simulink model "F16ASYM_ControlledFAST"  (R2012b)
settings: Solver=ode4  SolverMode=SingleTasking  StartTime=0.0  StopTime=inf  FixedStep=T_sim  RelTol=1e-3
InitFcn:
  | mex nlplantASYM.c
values from neighbouring files (symbols this model uses):
  T_sim = 0.02    [RUN_ME.m]
undefined symbols (not defined in the file or in its folder): B, dLEF, Earth, fi_flag_Simulink, k_B, latitude, longitude, m, m_B, Model_used_flag, rad, s, sigbuilder_block, trim_control, trim_state, trim_throttle, WGS84
libraries: F16_Actuator_Library x14, simulink_extras x9, aerolibatmos2 x3, aerolibtransform2 x3, aerolibfltsims x3, aerolibconvert2 x2, dspmtrx3 x1, qcatlib x1, aerolibasang x1, aerolibanimutils x1, aerolibconvert x1, aerolibobsolete x1
(part 1 of 2)
settings Model: SimulationMode=accelerator  Creator=David  LastModifiedBy=David
settings DataIOCC: SaveOutput=off  SignalLogging=off  DSMLogging=off  SaveTime=off

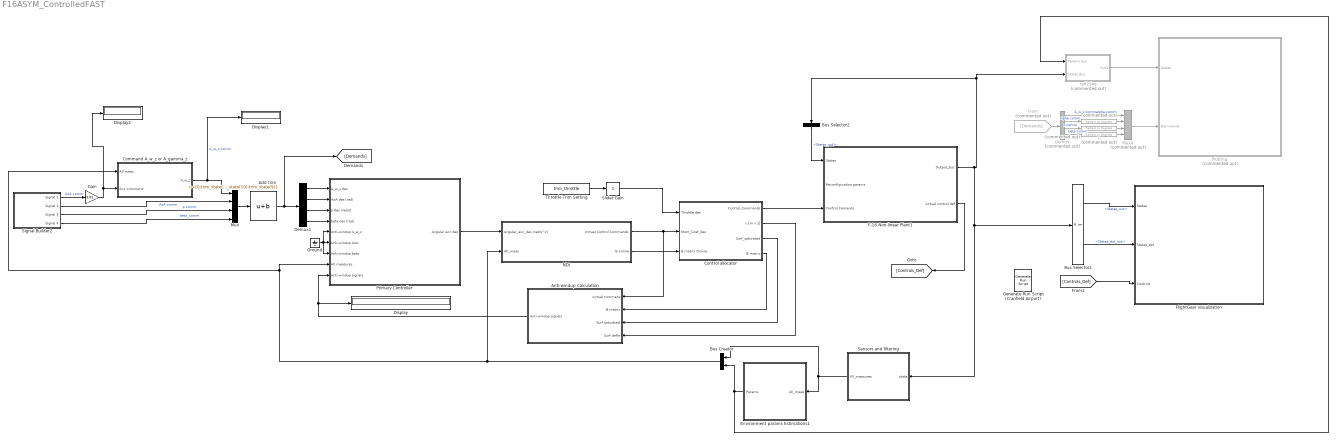
== system F16ASYM_ControlledFAST ==
  "  " : simulink_extras/Transformations/Radians to Degrees  Commented=on
  "  1" : simulink_extras/Transformations/Radians to Degrees  Commented=on
  "  2" : simulink_extras/Transformations/Radians to Degrees  Commented=on
  Add trim : Bias  Bias=[0;trim_state(8);trim_state(10);trim_state(9)]
  Anti-windup Calculation : Subsystem
  Bus Creator : BusCreator  Inputs=2
  Bus Selector1 : BusSelector  OutputSignals=States_out,States_dot_out
  Bus Selector2 : BusSelector  OutputSignals=States_out
  Command A_w_z or A_gamma_z : Subsystem  mask{Crit=A_w_z, Criteria=0}
      mask prompts: Crit "Commdn in:"
      mask init:
      | val = get_param(gcb,'MaskValues');
      | switch lower(val{1})
      |  case 'A_w_z'
      |      Criteria=0;
      |  case 'A_gamma_z'
      |      Criteria=1;
      | end
      mask TypeOptions Crit: A_w_z | A_gamma_z
      mask Display:
      | val = get_param(gcb,'MaskValues');
      | 
      | disp(['{\bf\fontsize{16}',upper(val{1}),'}'], 'texmode','on');
  Control allocator : Subsystem  RTWFcnName=abc  RTWFileName=asas  VariantObject=LinAndLin
      settings: RTWFcnNameOpts=User specified  RTWFileNameOpts=User specified
  Demux : Demux  Commented=on
  Demux1 : Demux
  Display : Display
  Display1 : Display
  Display2 : Display
  Environment params Estimations1 : Subsystem
      mask help: Simulink:masks:GenSFuncDesc_MD
      mask Help: eval('feval(''rtwprivate'',''rtwhelpview'',''rtw_sfcn_block'')');
  F-16 Non-linear Plant1 : Subsystem  Variant=on  OverrideUsingVariant=No Reconfigurable
      mask Display:
      | image(imread('f16.jpg'))
      | 
      | port_label('output', 1, 'Out_bus')
      | port_label('output', 2, 'Actual Control deflec')
      | 
      | port_label('input', 1, 'State_feedback')
      | port_label('input', 2, 'Reconfiguration params')
      | port_label('input', 3, 'Control_Commands')
      | 
      | % Variant dealing
      | ActiveVar = get_param(gcb,'activevariant');
      | 
      | 
      | disp(['{\bf\fontsize{16}',ActiveVar,'}'], 'texmode','on');
  FlightGear visualization : Subsystem  TreatAsAtomicUnit=on
      mask Display:
      | % disp('{\bf\fontsize{20} Flight Gear}', 'texmode','on');
      | image(imread('FG F16.jpg'))
      | % image(imread('FlightGear_logo.png'))
  From : From  Commented=on  GotoTag=Demands
  Gain : Gain  Gain=9.81
  Generate Run Script (Cranfield Airport) : aerolibfltsims/Generate Run Script  OutputFileName=runfg.bat  FlightGearBaseDirectory=C:\Program Files\FlightGear  GeometryModelName=f16  DestinationPort=5502  OriginAddress=127.0.0.1  OriginPort=5505  LocalAddress=127.0.0.1  AirportId=EGTC  RunwayId=1  InitialAltitude=trim_state(3)*3.2808399  InitialHeading=0  OffsetDistance=4.72  OffsetAzimuth=0  GenerateFile=off  Architecture=Win64  dataFlow=Send
  Ground : Ground
  Mux : Mux
  Mux4 : Mux  Commented=on
  NDI : Subsystem  RTWFcnName=abc  RTWFileName=asas  VariantObject=LinAndLin
      settings: RTWFcnNameOpts=User specified  RTWFileNameOpts=User specified
  Plotting : Subsystem  Commented=on
      mask Display:
      | disp('{\bf\fontsize{20} Plotting}', 'texmode','on');
      | % port_label('input', 1, 'States')
      | % port_label('input', 2, 'Demans')
  Primary Controller : Subsystem
      mask help: Simulink:masks:GenSFuncDesc_MD
      mask Help: eval('feval(''rtwprivate'',''rtwhelpview'',''rtw_sfcn_block'')');
  Sensors and filtering : Subsystem
  Signal Builder2 : Subsystem  Tag=STV Subsys  LoadFcn=sigbuilder_block('load');  StartFcn=sigbuilder_block('start');  StopFcn=sigbuilder_block('stop');  ClipboardFcn=sigbuilder_block('clipboard');  mask(Sigbuilder block){}
      mask help: Simulink:masks:SigbuilderBlock_MD
      mask init:
      | if ~strcmp(get_param(bdroot(gcbh),'SimulationStatus'),'stopped') tuvar = sigbuilder_block('maskInit'); end
      settings: CopyFcn=sigbuilder_block('copy');  DeleteFcn=sigbuilder_block('delete');  ModelCloseFcn=sigbuilder_block('modelClose');  PreSaveFcn=sigbuilder_block('preSave');  PauseFcn=sigbuilder_block('pause');  ContinueFcn=sigbuilder_block('continue');  NameChangeFcn=sigbuilder_block('namechange');  OpenFcn=sigbuilder_block('open',[6 28.5 1012.5 484.5 ]);  CloseFcn=sigbuilder_block('close');
      mask Display: plot(0, 0, 100, 100,[2, 2, 32, 32, 2], [68, 8, 8, 68, 68],[32, 2], [38, 38], [32, 19, 2],[53, 60, 44], [32, 17, 17, 2],[16, 16, 31, 31]);txt = getActiveGroup(gcbh);text(2, 100, txt,'verticalAlignment', 'top');
  Slider Gain : simulink/Math Operations/Slider Gain  low=0  gain=1  high=20
  Throttle Trim Setting : Constant  Value=trim_throttle
  rad2deg : Subsystem  Commented=on
  wires:
  rad2deg/1(Out1) -> Plotting/1(States)
  F-16 Non-linear Plant1/1(Output_bus) -> Bus Selector1/1, Sensors and filtering/1(state), Bus Selector2/1, rad2deg/2(States Bus)
  Bus Selector1/1 -> FlightGear visualization/1(States)  "<States_out>"
  Bus Selector1/2 -> FlightGear visualization/2(States_dot)  "<States_dot_out>"
  Control allocator/1(Control_Commands) -> F-16 Non-linear Plant1/3(Control Comands)
  From/1 -> Demux/1
  Sensors and filtering/1(All_measures) -> Environment params Estimations1/1(All_meas), Bus Creator/1
  Environment params Estimations1/1(Params) -> Bus Creator/2, rad2deg/1(Params bus)
  Bus Creator/1 -> NDI/2(All_meas), Primary Controller/8(All measures), Command A_w_z or A_gamma_z/1(All meas)
  Throttle Trim Setting/1 -> Slider Gain/1
  Demux/3 -> "  1"/1  "p comm"
  Demux/4 -> "  2"/1  "beta comm"
  Demux/2 -> "  "/1  "alpha comm"
  [Controls_Def] -> FlightGear visualization/3(Controls)
  F-16 Non-linear Plant1/2(Actual control def) -> [Controls_Def]
  Control allocator/2(u [m x 1]) -> Anti-windup Calculation/4(Surf defle)
  Control allocator/3(Surf_saturated) -> Anti-windup Calculation/3(Surf saturated)
  Control allocator/4(B matrix) -> Anti-windup Calculation/2(B matrix)
  NDI/1(Virtual Control Commands) -> Anti-windup Calculation/1(virtual commans), Control allocator/2(Mom_Coef_des)
  Anti-windup Calculation/1(Anti-windup signals) -> Primary Controller/9(Anti-windup signals), Display/1
  Primary Controller/1(Angular acc des) -> NDI/1(Angular_acc_des (rad/s^2))
  Ground/1 -> Primary Controller/7(Anti-windup beta), Primary Controller/6(Anti-windup AoA), Primary Controller/5(Anti-windup A_w_z)
  Mux/1 -> Add trim/1
  Demux1/3 -> Primary Controller/3(p des (rad/s))
  Demux1/4 -> Primary Controller/4(beta des (rad))
  Demux1/1 -> Primary Controller/1(A_w_z des)
  Mux4/1 -> Plotting/2(Demmands)
  Slider Gain/1 -> Control allocator/1(Throttle des)
  Bus Selector2/1 -> F-16 Non-linear Plant1/1(States)  "<States_out>"
  NDI/2(B online) -> Control allocator/3(B matrix Online)
  Add trim/1 -> [Demands], Demux1/1
  Demux1/2 -> Primary Controller/2(AoA des (rad))
  Signal Builder2/3(Signal 3) -> Mux/3  "p comm"
  Signal Builder2/2(Signal 2) -> Mux/2  "AoA comm"
  Command A_w_z or A_gamma_z/1(A_w_z) -> Display1/1, Mux/1  "A_w_z comm"
  Signal Builder2/4(Signal 4) -> Mux/4  "beta_comm"
  Demux/1 -> Mux4/1  "A_w_z commalpha comm"
  "  "/1 -> Mux4/2
  "  1"/1 -> Mux4/3
  "  2"/1 -> Mux4/4
  Signal Builder2/1(Signal 1) -> Gain/1  "AoA comm"
  Gain/1 -> Display2/1, Command A_w_z or A_gamma_z/2(Acc command)

== system F16ASYM_ControlledFAST/Anti-windup Calculation ==
  virtual commans : Inport
  B matrix : Inport  Port=2
  Surf saturated : Inport  Port=3
  Surf defle : Inport  Port=4
  Abs : Abs
  Add : Sum  Inputs=-+|
  Manual Switch : ManualSwitch  CurrentSetting=0
  Matrix Multiply : Product  Multiplication=Matrix(*)
  Matrix Multiply1 : Product
  Anti-windup signals : Outport
  wires:
  B matrix/1 -> Matrix Multiply/1
  Matrix Multiply/1 -> Add/2
  virtual commans/1 -> Add/1
  Add/1 -> Anti-windup signals/1
  Surf saturated/1 -> Abs/1
  Surf defle/1 -> Manual Switch/1, Matrix Multiply1/1
  Abs/1 -> Matrix Multiply1/2
  Manual Switch/1 -> Matrix Multiply/2
  Matrix Multiply1/1 -> Manual Switch/2

== system F16ASYM_ControlledFAST/Command A_w_z or A_gamma_z ==
  note: Pass this one if >0.5
  All meas : Inport
  Acc command : Inport  Port=2
  A_b : Product  Multiplication=Matrix(*)
  A_w : Product  Multiplication=Matrix(*)
  Bus Selector3 : BusSelector  OutputSignals=signal2.T_F_b->F_T,signal2.T_F_b->F_w
  Criteria : Constant  Value=Criteria
  Gain : Gain  Gain=[0,0,-1]
  Gain1 : Gain  Gain=-1
  Selector : Selector  InputPortWidth=3  IndexOptions=Index vector (dialog)  Indices=3  OutputSizes=1
  Switch : Switch  Threshold=0.5
  Transpose : dspmtrx3/Transpose  Hermitian=off  overflowFlag=off
  A_w_z : Outport
  wires:
  All meas/1 -> Bus Selector3/1
  Criteria/1 -> Switch/2
  Acc command/1 -> Switch/3, Gain/1
  Switch/1 -> A_w_z/1
  Bus Selector3/1 -> Transpose/1  "<T_F_b->F_T>"
  Transpose/1 -> A_b/1
  Gain/1 -> A_b/2
  Bus Selector3/2 -> A_w/1  "<T_F_b->F_w>"
  A_b/1 -> A_w/2
  A_w/1 -> Selector/1
  Selector/1 -> Gain1/1
  Gain1/1 -> Switch/1

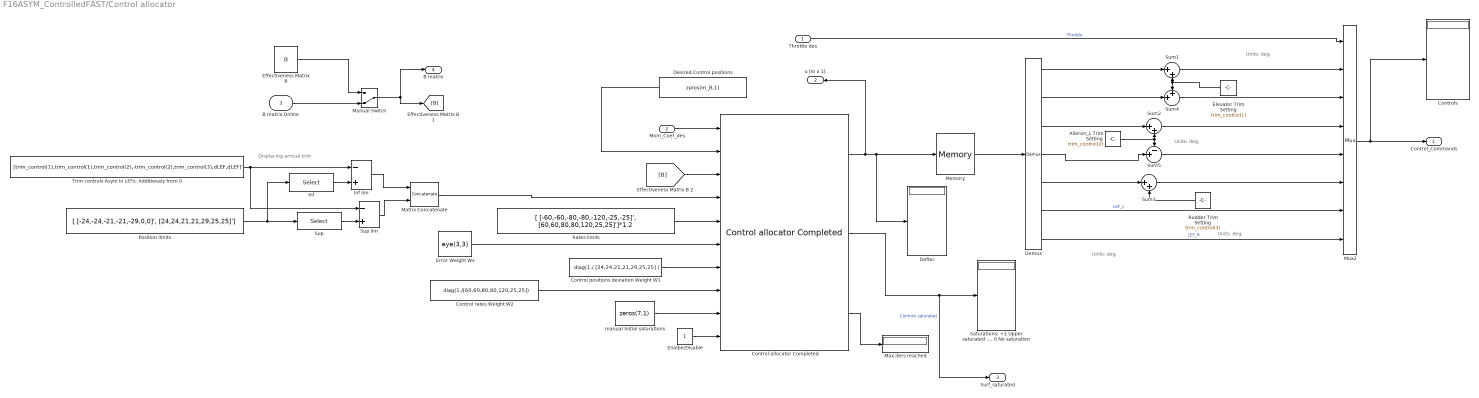
== system F16ASYM_ControlledFAST/Control allocator ==
  note: Displacing arroud trim
  note: Units: deg.
  note: Units: deg.
  note: Units: deg.
  note: Units: deg.
  Throttle des : Inport
  Mom_Coef_des : Inport  Port=2
  B matrix Online : Inport  Port=3
  Aileron_L Trim Setting : Constant  Value=trim_control(2)
  "Control allocator Completed " : qcatlib/Control allocator Completed   alg=WLS  CA_type=DYN  iter_max=10  gamma=1e6  k_B=3  m_B=7  T=T_sim  tol=1e-5
  Control positions deviation Weight W1 : Constant  Value=diag(1./ [24,24,21,21,29,25,25] )
  Control rates Weight W2 : Constant  Value=diag(1./[60,60,80,80,120,25,25])
  Controls : Display
  Deflec : Display
  Demux : Demux  Outputs=[1,1,1,1,1,1,1]
  Desired Control positions : Constant  Value=zeros(m_B,1)
  Effectiveness Matrix B : Constant  Value=B
  Elevator Trim Setting : Constant  Value=trim_control(1)  VectorParams1D=off
  Enalbe/Disable : Constant
  Error Weight Wv : Constant  Value=eye(3,3)
  Inf : Selector  NumberOfDimensions=2  InputPortWidth=3  IndexOptions=Index vector (dialog),Index vector (dialog)  Indices=[1:7],1  OutputSizes=1,1
  Inf lim : Sum  Inputs=-+
  Manual Switch : ManualSwitch  CurrentSetting=0
  Matrix Concatenate : Concatenate  Mode=Multidimensional array  ConcatenateDimension=2
  Max iters reached : Display
  Memory : Memory  X0=zeros(7,1)
  Mux2 : Mux  Inputs=8
  Position limits : Constant  Value=[ [-24,-24,-21,-21,-29,0,0]', [24,24,21,21,29,25,25]']
  Rates limits : Constant  Value=[ [-60,-60,-80,-80,-120,-25,-25]', [60,60,80,80,120,25,25]']*1.2
  Rudder Trim Setting : Constant  Value=trim_control(3)
  Saturations: +1 Upper saturated -1 Lower saturated 0 No saturation : Display
  Sum1 : Sum  Inputs=|++  SaturateOnIntegerOverflow=on  InputSameDT=on  OutDataTypeStr=Inherit: Same as first input
  Sum2 : Sum  Inputs=|++  SaturateOnIntegerOverflow=on  InputSameDT=on  OutDataTypeStr=Inherit: Same as first input
  Sum3 : Sum  Inputs=|++  SaturateOnIntegerOverflow=on  InputSameDT=on  OutDataTypeStr=Inherit: Same as first input
  Sum4 : Sum  Inputs=++|  SaturateOnIntegerOverflow=on  InputSameDT=on  OutDataTypeStr=Inherit: Same as first input
  Sum5 : Sum  Inputs=-+|  SaturateOnIntegerOverflow=on  InputSameDT=on  OutDataTypeStr=Inherit: Same as first input
  Sup : Selector  NumberOfDimensions=2  InputPortWidth=3  IndexOptions=Index vector (dialog),Index vector (dialog)  Indices=[1:7],2  OutputSizes=1,1
  Sup lim : Sum  Inputs=-+
  Trim controls Asym In LEFs: Additionaly from 0 : Constant  Value=[trim_control(1),trim_control(1),trim_control(2),-trim_control(2),trim_control(3),dLEF,dLEF]'
  manual Initial saturations : Constant  Value=zeros(7,1)
  Control_Commands : Outport
  u [m x 1] : Outport  Port=2
  Surf_saturated : Outport  Port=3
  B matrix : Outport  Port=4
  wires:
  Mom_Coef_des/1 -> "Control allocator Completed "/1
  Throttle des/1 -> Mux2/1  "Throttle"
  Mux2/1 -> Controls/1, Control_Commands/1
  Sum2/1 -> Mux2/4
  Sum3/1 -> Mux2/6
  Sum5/1 -> Mux2/5
  Aileron_L Trim Setting/1 -> Sum2/2, Sum5/1
  Sum1/1 -> Mux2/2
  Sum4/1 -> Mux2/3
  Demux/6 -> Mux2/7  "LEF_L"
  Demux/7 -> Mux2/8  "LEF_R"
  Demux/1 -> Sum1/1
  Demux/2 -> Sum4/2
  Demux/3 -> Sum2/1
  Demux/4 -> Sum5/2
  Elevator Trim Setting/1 -> Sum1/2, Sum4/1
  Rudder Trim Setting/1 -> Sum3/2
  Demux/5 -> Sum3/1
  "Control allocator Completed "/2 -> Surf_saturated/1, Saturations: +1 Upper saturated -1 Lower saturated 0 No saturation/1  "Controls saturated"
  Desired Control positions/1 -> "Control allocator Completed "/2
  Position limits/1 -> Inf/1, Sup/1
  Rates limits/1 -> "Control allocator Completed "/5
  Error Weight Wv/1 -> "Control allocator Completed "/6
  Control positions deviation Weight W1/1 -> "Control allocator Completed "/7
  Control rates Weight W2/1 -> "Control allocator Completed "/8
  Sup/1 -> Sup lim/2
  Trim controls Asym In LEFs: Additionaly from 0/1 -> Sup lim/1, Inf lim/1
  Inf/1 -> Inf lim/2
  Matrix Concatenate/1 -> "Control allocator Completed "/4
  Inf lim/1 -> Matrix Concatenate/1
  Sup lim/1 -> Matrix Concatenate/2
  [B] -> "Control allocator Completed "/3
  "Control allocator Completed "/3 -> Max iters reached/1
  manual Initial saturations/1 -> "Control allocator Completed "/9
  Enalbe/Disable/1 -> "Control allocator Completed "/10
  "Control allocator Completed "/1 -> u [m x 1]/1, Memory/1, Deflec/1
  Memory/1 -> Demux/1
  B matrix Online/1 -> Manual Switch/2
  Effectiveness Matrix B/1 -> Manual Switch/1
  Manual Switch/1 -> [B], B matrix/1

== system F16ASYM_ControlledFAST/Environment params Estimations1 ==
  All_meas : Inport
  Environment params Estimations_sfcn : S-Function  FunctionName=Environment_sf  SFunctionModules=""  EnableBusSupport=off  mask{rtw_sf_name=Environment_sf, showVar=off}
      mask prompts: rtw_sf_name "Simulink:masks:GenSFuncName_MP"; showVar "Simulink:masks:GenSFuncShowModuleList_MP"
      mask help: Simulink:masks:GenSFuncDesc_MD
      mask init:
      | displist = '';
      | if ~strcmp(get_param(gcb, 'FunctionName'), rtw_sf_name);
      |   set_param(gcb, 'FunctionName', rtw_sf_name);
      | end
      | % Check if we are generating code
      | rtw_mode = false;
      | if strcmpi(get_param(bdroot(gcb),'SimulationStatus'),'Initializing')
      | 	rtw_mode = strcmpi(get_param(bdroot(gcb),'BuildingRTWCode'),'on') && ...
      | 		~strcmpi(get_param(bdroot(gcb),'TargetStyle'),'SimulationTarget');
      | end
      | if showVar || rtw_mode
      | 	if exist('rtwsfunc') == 2 | exist('rtwsfunc') == 6
      | 		tmplist = rtwsfunc(rtw_sf_name,gcb);
      | 		tmplist = DAStudio.message('Simulink:masks:GenSFuncListOfModules_IC', tmplist);
      | 	elseif showVar
      | 		tmplist1 = DAStudio.message('Simulink:masks:GenSFuncListOfModules_IC', '');
      |         tmplist2 = DAStudio.message('Simulink:masks:GenSFuncNotLicensed_IC');
      |         tmplist = [tmplist1 tmplist2];
      |  	end
      | end
      | if showVar
      |   displist = tmplist;
      | end
      settings: CopyFcn=|
      | if ~strcmp(get_param(gcb,'Linkstatus'),'none') && ...
      | ~strcmp(get_param(gcb,'Linkstatus'),'implicit')
      |   set_param(gcb,'LinkStatus','none');
      | end
      mask Help: eval('feval(''rtwprivate'',''rtwhelpview'',''rtw_sfcn_block'')');
      mask Display:
      | port_label('input',1,'Alt meas (m)');
      | port_label('input',2,'V_TAS (m/s)');
      | port_label('input',3,'AoA meas (rad)');
      | port_label('input',4,'SS meas (rad)');
      | port_label('input',5,'omega_b meas (rad/s)');
      | port_label('input',6,'Euler meas (rad)');
      | port_label('input',7,'an_b_CG meas (m/s^2)');
      | port_label('input',8,'Throttle_meas');
      | port_label('output',1,'q (Pa)');
      | port_label('output',2,'T_F_b->F_T');
      | port_label('output',3,'T_F_b->F_w');
      | port_label('output',4,'A_w_CG');
      | port_label('output',5,'A_b_CG');
  __InputSSForSFun__ : Subsystem
  __OutputSSForSFun__ : Subsystem
  Params : Outport
  wires:
  All_meas/1 -> __InputSSForSFun__/1(All_meas)
  __InputSSForSFun__/1(__UniqueOutportName__1__) -> Environment params Estimations_sfcn/1
  __InputSSForSFun__/2(__UniqueOutportName__2__) -> Environment params Estimations_sfcn/2
  __InputSSForSFun__/3(__UniqueOutportName__3__) -> Environment params Estimations_sfcn/3
  __InputSSForSFun__/4(__UniqueOutportName__4__) -> Environment params Estimations_sfcn/4
  __InputSSForSFun__/5(__UniqueOutportName__5__) -> Environment params Estimations_sfcn/5
  __InputSSForSFun__/6(__UniqueOutportName__6__) -> Environment params Estimations_sfcn/6
  __InputSSForSFun__/7(__UniqueOutportName__7__) -> Environment params Estimations_sfcn/7
  __InputSSForSFun__/8(__UniqueOutportName__8__) -> Environment params Estimations_sfcn/8
  Environment params Estimations_sfcn/1 -> __OutputSSForSFun__/1(__UniqueInportName__1__)
  Environment params Estimations_sfcn/2 -> __OutputSSForSFun__/2(__UniqueInportName__2__)
  Environment params Estimations_sfcn/3 -> __OutputSSForSFun__/3(__UniqueInportName__3__)
  Environment params Estimations_sfcn/4 -> __OutputSSForSFun__/4(__UniqueInportName__4__)
  Environment params Estimations_sfcn/5 -> __OutputSSForSFun__/5(__UniqueInportName__5__)
  __OutputSSForSFun__/1(Params) -> Params/1

== system F16ASYM_ControlledFAST/F-16 Non-linear Plant1 ==
  States : Inport
  Reconfiguration params : Inport  Port=2
  Control Comands : Inport  Port=3
  SYM and ASYM model: No reconfigurable : Subsystem  VariantObject=No Reconfigurable
  SYM and ASYM model: RECONFIGURABLE : Subsystem  VariantObject=Reconfigurable
  Output_bus : Outport
  Actual control def : Outport  Port=2

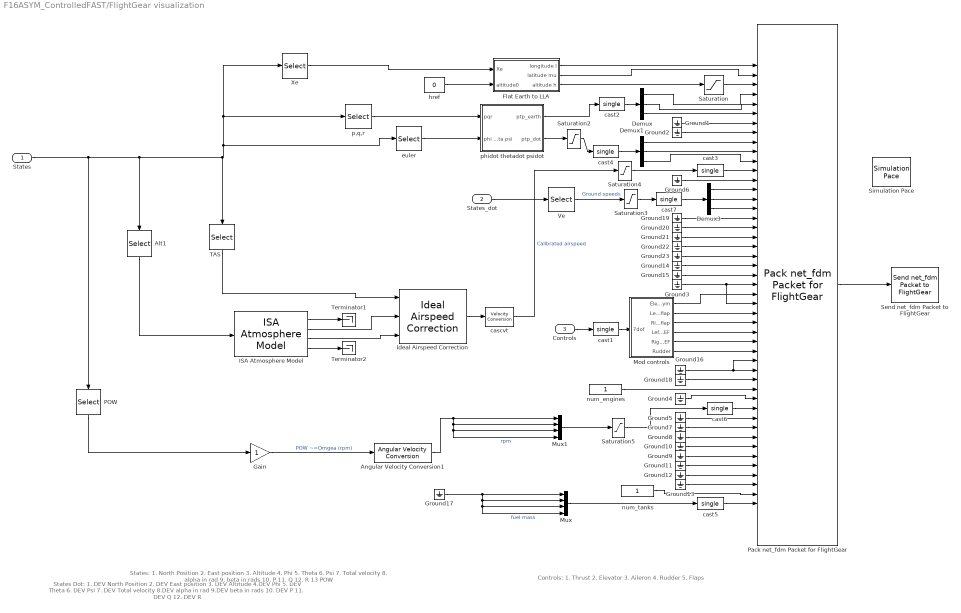
== system F16ASYM_ControlledFAST/FlightGear visualization ==
  note: States Dot:
      | 1. DEV North Position
      | 2. DEV East position
      | 3. DEV Altitude
      | 4.DEV  Phi
      | 5. DEV Theta
      | 6. DEV Psi
      | 7. DEV Total velocity
      | 8.DEV alpha in rad
      | 9.DEV  beta in rads
      | 10. DEV P
      | 11. DEV Q
      | 12. DEV R
  note: States:
      | 1. North Position
      | 2. East position
      | 3. Altitude
      | 4. Phi
      | 5. Theta
      | 6. Psi
      | 7. Total velocity
      | 8. alpha in rad
      | 9. beta in rads
      | 10. P
      | 11. Q
      | 12. R
      | 13 POW
  note: Controls:
      | 1. Thrust
      | 2. Elevator
      | 3. Aileron
      | 4. Rudder
      | 5. Flaps
  States : Inport
  States_dot : Inport  Port=2
  Controls : Inport  Port=3
  Alt1 : Selector  InputPortWidth=13  IndexOptions=Index vector (dialog)  Indices=3  OutputSizes=1
  Angular Velocity Conversion1 : aerolibconvert2/Angular Velocity Conversion  IU=rad/s  OU=rpm
  Demux : Demux  Outputs=3
  Demux1 : Demux  Outputs=3
  Demux3 : Demux  Outputs=3
  Flat Earth to LLA : Subsystem
  Gain : Gain
  Ground{1..23} (23 alike) : Ground
  ISA Atmosphere Model : aerolibatmos2/ISA Atmosphere Model  custom=off  g=9.80665  gamma=1.4  R=287.0531  L=0.0065  h_trop=11000  h_strat=20000  rho0=1.225  P0=101325  T0=288.15
  Ideal Airspeed Correction : aerolibasang/Ideal Airspeed Correction  units=Metric (MKS)  vel_in=TAS  vel_out_tas=CAS  vel_out_eas=CAS  vel_out_cas=TAS  action=Warning
  Mod controls : Subsystem
  Mux : Mux
  Mux1 : Mux
  POW : Selector  InputPortWidth=13  IndexOptions=Index vector (dialog)  Indices=13  OutputSizes=1
  Pack net_fdm Packet for FlightGear : aerolibfltsims/Pack net_fdm Packet for FlightGear  FlightGearVersion=v2.0  ShowPositionAttitudeInputs=on  ShowVelocityAccelerationInputs=on  ShowControlSurfacePositionInputs=on  ShowEngineFuelInputs=on  ShowLandingGearInputs=off  ShowEnvironmentInputs=off  SampleTime=-1
      settings: AttributesFormatString=FG VERSION: %<FlightGearVersion>
  Saturation : Saturate  UpperLimit=1e8  LowerLimit=-1e5
  Saturation2 : Saturate  UpperLimit=1e3  LowerLimit=-1e3
  Saturation3 : Saturate  UpperLimit=1e4  LowerLimit=-1e4
  Saturation4 : Saturate  UpperLimit=1e4  LowerLimit=-1e4
  Saturation5 : Saturate  UpperLimit=1e6  LowerLimit=0
  Send net_fdm Packet to FlightGear : aerolibfltsims/Send net_fdm Packet to FlightGear  DestinationIpAddress=127.0.0.1  DestinationPort=5502  LocalIpPort=-1  varLen=off  SampleTime=-1
  Simulation Pace : aerolibanimutils/Simulation Pace  SimulationPace=1  SleepMode=MATLAB Thread  OutputPaceError=off  SampleTime=4*T_sim
      settings: AttributesFormatString=%<SimulationPace> sec/sec
  TAS : Selector  InputPortWidth=13  IndexOptions=Index vector (dialog)  Indices=7  OutputSizes=1
  Terminator1 : Terminator
  Terminator2 : Terminator
  Ve : Selector  InputPortWidth=13  IndexOptions=Index vector (dialog)  Indices=[1:3]  OutputSizes=1
  Xe : Selector  InputPortWidth=13  IndexOptions=Index vector (dialog)  Indices=[1:3]  OutputSizes=1
  cascvt : aerolibconvert/Velocity Conversion  IU=m/s  OU=kts
  cast{1..7} (7 alike) : DataTypeConversion  OutDataTypeStr=single  SaturateOnIntegerOverflow=on
  euler : Selector  InputPortWidth=13  IndexOptions=Index vector (dialog)  Indices=[4:6]  OutputSizes=1
  href : Constant  Value=0  VectorParams1D=off
  num_engines : Constant  OutDataTypeStr=uint32
  num_tanks : Constant  OutDataTypeStr=uint32
  p,q,r : Selector  InputPortWidth=13  IndexOptions=Index vector (dialog)  Indices=[10:12]  OutputSizes=1
  phidot thetadot psidot : Subsystem
  wires:
  Pack net_fdm Packet for FlightGear/1 -> Send net_fdm Packet to FlightGear/1
  Ground3/1 -> Pack net_fdm Packet for FlightGear/26, Pack net_fdm Packet for FlightGear/24
  Demux1/3 -> Pack net_fdm Packet for FlightGear/11
  Demux1/2 -> Pack net_fdm Packet for FlightGear/10
  Demux1/1 -> Pack net_fdm Packet for FlightGear/9
  Ground2/1 -> Pack net_fdm Packet for FlightGear/8
  Ground1/1 -> Pack net_fdm Packet for FlightGear/7
  Demux/3 -> Pack net_fdm Packet for FlightGear/6
  Demux/2 -> Pack net_fdm Packet for FlightGear/5
  Demux/1 -> Pack net_fdm Packet for FlightGear/4
  Ground6/1 -> Pack net_fdm Packet for FlightGear/13
  ISA Atmosphere Model/2 -> Ideal Airspeed Correction/2
  phidot thetadot psidot/2(ptp_dot) -> Saturation2/1
  phidot thetadot psidot/1(ptp_earth) -> cast2/1
  cast3/1 -> Pack net_fdm Packet for FlightGear/12
  cascvt/1 -> Saturation4/1  "Calibrated airspeed"
  Ideal Airspeed Correction/1 -> cascvt/1
  Ground15/1 -> Pack net_fdm Packet for FlightGear/23
  Ground14/1 -> Pack net_fdm Packet for FlightGear/22
  Ground23/1 -> Pack net_fdm Packet for FlightGear/21
  Ground22/1 -> Pack net_fdm Packet for FlightGear/20
  Ground21/1 -> Pack net_fdm Packet for FlightGear/19
  Ground20/1 -> Pack net_fdm Packet for FlightGear/18
  Ground19/1 -> Pack net_fdm Packet for FlightGear/17
  href/1 -> Flat Earth to LLA/2(altitude0)
  Flat Earth to LLA/3(altitude h) -> Saturation/1
  States/1 -> p,q,r/1, Xe/1, euler/1, TAS/1, Alt1/1, POW/1
  Flat Earth to LLA/1(longitude l) -> Pack net_fdm Packet for FlightGear/1
  Flat Earth to LLA/2(latitude mu) -> Pack net_fdm Packet for FlightGear/2
  Demux3/1 -> Pack net_fdm Packet for FlightGear/14
  Demux3/2 -> Pack net_fdm Packet for FlightGear/15
  Demux3/3 -> Pack net_fdm Packet for FlightGear/16
  Ve/1 -> Saturation3/1  "Ground speeds"
  cast2/1 -> Demux/1
  cast4/1 -> Demux1/1
  cast5/1 -> Pack net_fdm Packet for FlightGear/47
  cast6/1 -> Pack net_fdm Packet for FlightGear/37
  num_tanks/1 -> Pack net_fdm Packet for FlightGear/46
  ISA Atmosphere Model/1 -> Terminator1/1
  ISA Atmosphere Model/4 -> Terminator2/1
  ISA Atmosphere Model/3 -> Ideal Airspeed Correction/3
  Alt1/1 -> ISA Atmosphere Model/1
  Ground17/1 -> Mux/2, Mux/3, Mux/4, Mux/1  "fuel mass"
  Mux/1 -> cast5/1
  Gain/1 -> Angular Velocity Conversion1/1  "POW ~=Omgea (rpm)"
  Mux1/1 -> Saturation5/1
  cast7/1 -> Demux3/1
  Angular Velocity Conversion1/1 -> Mux1/2, Mux1/3, Mux1/4, Mux1/1  "rpm"
  Saturation/1 -> Pack net_fdm Packet for FlightGear/3
  Saturation2/1 -> cast4/1
  Saturation3/1 -> cast7/1
  Saturation4/1 -> cast3/1
  Saturation5/1 -> cast6/1
  States_dot/1 -> Ve/1
  Ground5/1 -> Pack net_fdm Packet for FlightGear/38
  Ground7/1 -> Pack net_fdm Packet for FlightGear/39
  Ground8/1 -> Pack net_fdm Packet for FlightGear/40
  Ground10/1 -> Pack net_fdm Packet for FlightGear/41
  Ground9/1 -> Pack net_fdm Packet for FlightGear/42
  Ground11/1 -> Pack net_fdm Packet for FlightGear/43
  Ground12/1 -> Pack net_fdm Packet for FlightGear/44
  Ground13/1 -> Pack net_fdm Packet for FlightGear/45
  Ground4/1 -> Pack net_fdm Packet for FlightGear/36
  num_engines/1 -> Pack net_fdm Packet for FlightGear/35
  Controls/1 -> cast1/1
  Ground18/1 -> Pack net_fdm Packet for FlightGear/34
  Ground16/1 -> Pack net_fdm Packet for FlightGear/32, Pack net_fdm Packet for FlightGear/33
  Xe/1 -> Flat Earth to LLA/1(Xe)
  euler/1 -> phidot thetadot psidot/2(phi theta psi)
  TAS/1 -> Ideal Airspeed Correction/1
  p,q,r/1 -> phidot thetadot psidot/1(pqr)
  POW/1 -> Gain/1
  cast1/1 -> Mod controls/1("7dof ")
  Mod controls/1(Elevator Sym) -> Pack net_fdm Packet for FlightGear/25
  Mod controls/2(Left flap) -> Pack net_fdm Packet for FlightGear/27
  Mod controls/3(Right flap) -> Pack net_fdm Packet for FlightGear/28
  Mod controls/4(Left LEF) -> Pack net_fdm Packet for FlightGear/29
  Mod controls/5(Right LEF) -> Pack net_fdm Packet for FlightGear/30
  Mod controls/6(Rudder) -> Pack net_fdm Packet for FlightGear/31

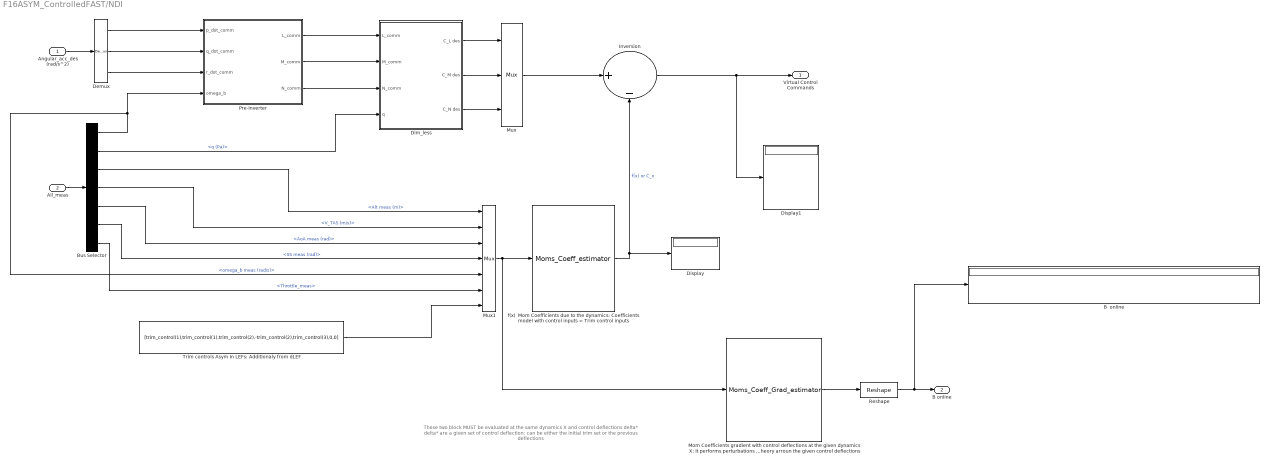
== system F16ASYM_ControlledFAST/NDI ==
  note: These two block MUST be evaluated at the same dynamics X
      | and control deflections delta*
      |
      |
      | delta* are a given set of control deflection: can be either the initial trim set
      | or the previous deflections
  Angular_acc_des (rad/s^2) : Inport
  All_meas : Inport  Port=2
  B  online : Display
  Bus Selector : BusSelector  OutputSignals=signal1.omega_b meas (rad/s),signal2.q (Pa),signal1.Alt meas (m),signal1.V_TAS (m/s),signal1.AoA meas (rad),signal1.SS meas (rad),signal1.Throttle_meas
  Demux : Demux  Outputs=3
  Dim_less : Subsystem
  Display : Display
  Display1 : Display
  Inversion : Sum  Inputs=|+-
  Mom Coefficients gradient with control deflections at the given dynamics X: It performs perturbations theory arroun the given control deflections : MATLABFcn  MATLABFcn=Moms_Coeff_Grad_estimator  OutputDimensions=21  OutputSignalType=real
  Mux : Mux  Inputs=3
  Mux1 : Mux  Inputs=7
  Pre-Inverter : MATLAB Function  TreatAsAtomicUnit=on
  Reshape : Reshape  OutputDimensionality=Customize  OutputDimensions=[k_B,m_B]
  Trim controls Asym In LEFs: Additionaly from dLEF : Constant  Value=[trim_control(1),trim_control(1),trim_control(2),-trim_control(2),trim_control(3),0,0]
  f(x)  Mom Coefficients due to the dynamics: Coefficients model with control inputs = Trim control inputs : MATLABFcn  MATLABFcn=Moms_Coeff_estimator  OutputDimensions=3  OutputSignalType=real
  Virtual Control Commands : Outport
  B online : Outport  Port=2
  wires:
  Inversion/1 -> Display1/1, Virtual Control Commands/1
  Bus Selector/1 -> Pre-Inverter/4(omega_b), Mux1/5  "<omega_b meas (rad/s)>"
  Angular_acc_des (rad/s^2)/1 -> Demux/1
  Demux/2 -> Pre-Inverter/2(q_dot_comm)
  Demux/3 -> Pre-Inverter/3(r_dot_comm)
  Demux/1 -> Pre-Inverter/1(p_dot_comm)
  All_meas/1 -> Bus Selector/1
  Bus Selector/2 -> Dim_less/4(q)  "<q (Pa)>"
  Pre-Inverter/1(L_comm) -> Dim_less/1(L_comm)
  Pre-Inverter/2(M_comm) -> Dim_less/2(M_comm)
  Pre-Inverter/3(N_comm) -> Dim_less/3(N_comm)
  Dim_less/1(C_L des) -> Mux/1
  Dim_less/2(C_M des) -> Mux/2
  Dim_less/3(C_N des) -> Mux/3
  f(x)  Mom Coefficients due to the dynamics: Coefficients model with control inputs = Trim control inputs/1 -> Inversion/2, Display/1  "f(x) or C_x"
  Bus Selector/3 -> Mux1/1  "<Alt meas (m)>"
  Bus Selector/4 -> Mux1/2  "<V_TAS (m/s)>"
  Bus Selector/5 -> Mux1/3  "<AoA meas (rad)>"
  Bus Selector/6 -> Mux1/4  "<SS meas (rad)>"
  Trim controls Asym In LEFs: Additionaly from dLEF/1 -> Mux1/7
  Mux1/1 -> f(x)  Mom Coefficients due to the dynamics: Coefficients model with control inputs = Trim control inputs/1, Mom Coefficients gradient with control deflections at the given dynamics X: It performs perturbations theory arroun the given control deflections/1
  Bus Selector/7 -> Mux1/6  "<Throttle_meas>"
  Mux/1 -> Inversion/1
  Mom Coefficients gradient with control deflections at the given dynamics X: It performs perturbations theory arroun the given control deflections/1 -> Reshape/1
  Reshape/1 -> B  online/1, B online/1

== system F16ASYM_ControlledFAST/Plotting ==
  States : Inport
  Demmands : Inport  Port=2
  Demux : Demux
  Demux1 : Demux  Outputs=20
  Mux{1..4} (4 alike) : Mux  Inputs=2
  Responses and commands : Scope  NumInputPorts=5
      settings: ShowLegends=on  TimeRange=10  YMin=-0.15~3.875~-0.00015~-0.343~159.35  YMax=0.45~4.2~0.00015~-0.3405~159.95  SaveName=ScopeData2  Decimation=2
  Scope{,1,3..4} (4 alike) : Scope  NumInputPorts=3
      Scope settings: YMin=12100~6e-11~13235  YMax=13700~8.75e-11~13320  Decimation=20
      Scope1 settings: TimeRange=10  YMin=202.5~-10~13  YMax=232.5~12.5~26  Decimation=2  SampleTime=0.001
      Scope3 settings: TimeRange=10  YMin=-3~-0.04~-3  YMax=7~0.04~9  SaveName=ScopeData3  Decimation=2
      Scope4 settings: YMin=-5~-5~-5  YMax=5~5~5  SaveName=ScopeData4  Decimation=20
  Scope5 : Scope  NumInputPorts=4
      settings: YMin=-5~-5~-5~-5  YMax=5~5~5~5  SaveName=ScopeData5  Decimation=20
  wires:
  Demux1/1 -> Scope/1  "npos   (m)"
  Demux1/2 -> Scope/2  "epos   (m)"
  Demux1/3 -> Scope/3  "alt   (m)"
  Demux1/5 -> Scope1/2  "theta   (deg)"
  Demux1/6 -> Scope1/3  "psi  (deg)"
  Demux1/7 -> Responses and commands/5  "TAS   (m/s)"
  Demux1/8 -> Mux1/2  "alpha( deg)"
  Demux1/9 -> Mux3/2  "beta  (deg)"
  Demux1/10 -> Scope3/1, Mux2/2  "p   (deg/s)"
  Demux1/11 -> Scope3/2  "q   (deg/s)"
  Demux1/12 -> Scope3/3  "r   (deg/s)"
  Demux1/14 -> Scope4/1  "nx (g)"
  Demux1/15 -> Scope4/2  "ny (g)"
  Demux1/16 -> Scope4/3  "nz (g)"
  Demux1/4 -> Scope1/1  "phi   (deg)"
  Demux1/17 -> Scope5/2  "mach"
  Demux1/18 -> Scope5/3  "qbar (Pa"
  Demux1/19 -> Scope5/4  "ps (Pa)"
  States/1 -> Demux1/1
  Demux1/13 -> Scope5/1  "pow"
  Demmands/1 -> Demux/1
  Mux1/1 -> Responses and commands/2
  Mux2/1 -> Responses and commands/3
  Mux3/1 -> Responses and commands/4
  Demux/2 -> Mux1/1  "alpha comm"
  Demux/3 -> Mux2/1  "p comm"
  Demux/4 -> Mux3/1  "beta comm"
  Mux4/1 -> Responses and commands/1
  Demux/1 -> Mux4/1  "A_w_z comm"
  Demux1/20 -> Mux4/2  "A_w_z"

== system F16ASYM_ControlledFAST/Primary Controller ==
  A_w_z des : Inport
  AoA des (rad) : Inport  Port=2
  p des (rad/s) : Inport  Port=3
  beta des (rad) : Inport  Port=4
  Anti-windup A_w_z : Inport  Port=5
  Anti-windup AoA : Inport  Port=6
  Anti-windup beta : Inport  Port=7
  All measures : Inport  Port=8
  Anti-windup signals : Inport  Port=9
  Primary Controller_sfcn : S-Function  FunctionName=Primary_sf  SFunctionModules=""  EnableBusSupport=off  mask{rtw_sf_name=Primary_sf, showVar=off}
      mask prompts: rtw_sf_name "Simulink:masks:GenSFuncName_MP"; showVar "Simulink:masks:GenSFuncShowModuleList_MP"
      mask help: Simulink:masks:GenSFuncDesc_MD
      mask init: same as F16ASYM_ControlledFAST/Environment params Estimations1/Environment params Estimations_sfcn
      settings: CopyFcn=|
      | if ~strcmp(get_param(gcb,'Linkstatus'),'none') && ...
      | ~strcmp(get_param(gcb,'Linkstatus'),'implicit')
      |   set_param(gcb,'LinkStatus','none');
      | end
      mask Help: eval('feval(''rtwprivate'',''rtwhelpview'',''rtw_sfcn_block'')');
      mask Display:
      | port_label('input',1,'A_w_z des');
      | port_label('input',2,'AoA des (rad)');
      | port_label('input',3,'p des (rad/s)');
      | port_label('input',4,'beta des (rad)');
      | port_label('input',5,'Anti-windup A_w_z');
      | port_label('input',6,'Anti-windup AoA');
      | port_label('input',7,'Anti-windup beta');
      | port_label('input',8,'Alt meas (m)');
      | port_label('input',9,'V_TAS (m/s)');
      | port_label('input',10,'AoA meas (rad)');
      | port_label('input',11,'SS meas (rad)');
      | port_label('input',12,'omega_b meas (rad/s)');
      | port_label('input',13,'Euler meas (rad)');
      | port_label('input',14,'an_b_CG meas (m/s^2)');
      | port_label('input',15,'Throttle_meas');
      | port_label('input',16,'q (Pa)');
      | port_label('input',17,'T_F_b->F_T');
      | port_label('input',18,'T_F_b->F_w');
      | port_label('input',19,'A_w_CG');
      | port_label('input',20,'A_b_CG');
      | port_label('input',21,'Anti-windup signals');
      | port_label('output',1,'Angular acc des');
  __InputSSForSFun__ : Subsystem
  __OutputSSForSFun__ : Subsystem
  Angular acc des : Outport
  wires:
  A_w_z des/1 -> __InputSSForSFun__/1(A_w_z des)
  AoA des (rad)/1 -> __InputSSForSFun__/2(AoA des (rad))
  p des (rad/s)/1 -> __InputSSForSFun__/3(p des (rad/s))
  beta des (rad)/1 -> __InputSSForSFun__/4(beta des (rad))
  Anti-windup A_w_z/1 -> __InputSSForSFun__/5(Anti-windup A_w_z)
  Anti-windup AoA/1 -> __InputSSForSFun__/6(Anti-windup AoA)
  Anti-windup beta/1 -> __InputSSForSFun__/7(Anti-windup beta)
  All measures/1 -> __InputSSForSFun__/8(All measures)
  Anti-windup signals/1 -> __InputSSForSFun__/9(Anti-windup signals)
  __InputSSForSFun__/1(__UniqueOutportName__1__) -> Primary Controller_sfcn/1
  __InputSSForSFun__/2(__UniqueOutportName__2__) -> Primary Controller_sfcn/2
  __InputSSForSFun__/3(__UniqueOutportName__3__) -> Primary Controller_sfcn/3
  __InputSSForSFun__/4(__UniqueOutportName__4__) -> Primary Controller_sfcn/4
  __InputSSForSFun__/5(__UniqueOutportName__5__) -> Primary Controller_sfcn/5
  __InputSSForSFun__/6(__UniqueOutportName__6__) -> Primary Controller_sfcn/6
  __InputSSForSFun__/7(__UniqueOutportName__7__) -> Primary Controller_sfcn/7
  __InputSSForSFun__/8(__UniqueOutportName__8__) -> Primary Controller_sfcn/8
  __InputSSForSFun__/9(__UniqueOutportName__9__) -> Primary Controller_sfcn/9
  __InputSSForSFun__/10(__UniqueOutportName__10__) -> Primary Controller_sfcn/10
  __InputSSForSFun__/11(__UniqueOutportName__11__) -> Primary Controller_sfcn/11
  __InputSSForSFun__/12(__UniqueOutportName__12__) -> Primary Controller_sfcn/12
  __InputSSForSFun__/13(__UniqueOutportName__13__) -> Primary Controller_sfcn/13
  __InputSSForSFun__/14(__UniqueOutportName__14__) -> Primary Controller_sfcn/14
  __InputSSForSFun__/15(__UniqueOutportName__15__) -> Primary Controller_sfcn/15
  __InputSSForSFun__/16(__UniqueOutportName__16__) -> Primary Controller_sfcn/16
  __InputSSForSFun__/17(__UniqueOutportName__17__) -> Primary Controller_sfcn/17
  __InputSSForSFun__/18(__UniqueOutportName__18__) -> Primary Controller_sfcn/18
  __InputSSForSFun__/19(__UniqueOutportName__19__) -> Primary Controller_sfcn/19
  __InputSSForSFun__/20(__UniqueOutportName__20__) -> Primary Controller_sfcn/20
  __InputSSForSFun__/21(__UniqueOutportName__21__) -> Primary Controller_sfcn/21
  Primary Controller_sfcn/1 -> __OutputSSForSFun__/1(__UniqueInportName__1__)
  __OutputSSForSFun__/1(Angular acc des) -> Angular acc des/1

== system F16ASYM_ControlledFAST/Sensors and filtering ==
  note: This is measured load factor
  note: There should be noise here in the midle
  state : Inport
  Bus Creator : BusCreator  Inputs=8
  Bus Selector2 : BusSelector  OutputSignals=X_e,TAS,alpha;beta,p;q;r,euler,an_b_CG,Throttle
  Demux : Demux  Outputs=3
  Demux1 : Demux  Outputs=2
  Gain{,1..4} (5 alike) : Gain
  Terminator : Terminator
  Terminator1 : Terminator
  All_measures : Outport
  wires:
  state/1 -> Bus Selector2/1
  Bus Selector2/1 -> Demux/1  "<X_e>"
  Demux/3 -> Bus Creator/1  "Alt meas (m)"
  Demux/1 -> Terminator/1
  Demux/2 -> Terminator1/1
  Bus Selector2/2 -> Gain/1  "<TAS>"
  Bus Selector2/3 -> Demux1/1  "<alpha;beta>"
  Demux1/1 -> Bus Creator/3  "AoA meas (rad)"
  Demux1/2 -> Bus Creator/4  "SS meas (rad)"
  Bus Selector2/4 -> Gain1/1  "<p;q;r>"
  Bus Selector2/5 -> Gain2/1  "<euler>"
  Bus Selector2/6 -> Gain3/1  "<an_b_CG>"
  Gain/1 -> Bus Creator/2  "V_TAS (m/s)"
  Gain1/1 -> Bus Creator/5  "omega_b meas (rad/s)"
  Gain2/1 -> Bus Creator/6  "Euler meas (rad)"
  Gain3/1 -> Bus Creator/7  "an_b_CG meas (m/s^2)"
  Bus Creator/1 -> All_measures/1
  Bus Selector2/7 -> Gain4/1  "<Throttle>"
  Gain4/1 -> Bus Creator/8  "Throttle_meas"

== system F16ASYM_ControlledFAST/Signal Builder2 ==
  Demux : Demux  Tag=STV Demux
  FromWs : FromWorkspace  Tag=STV FromWs  VariableName=tuvar  SampleTime=0
      SigBuilderData=|
      | common.afterFinalStr = 'Extrapolate'
      | common.sampleTime = 0
      | dataSet.timeRange = [0 10]
      | dataSet.name = 'Group 1'
      | sbobj.Groups.Name = 'Group 1'
      | sbobj.Groups.Signals(1).Name = 'Signal 1'
      | sbobj.Groups.Signals(1).XData = [0 1 1 8.07 8.07 10]
      | sbobj.Groups.Signals(1).YData = [0 0 -0.23 0.32 0.03 0.03]
      | sbobj.Groups.Signals(2).Name = 'Signal 2'
      | sbobj.Groups.Signals(2).XData = [0 10]
      | sbobj.Groups.Signals(2).YData = [0 0]
      | sbobj.Groups.Signals(3).Name = 'Signal 3'
      | sbobj.Groups.Signals(3).XData = [0 10]
      | sbobj.Groups.Signals(3).YData = [0 0]
      | sbobj.Groups.Signals(4).Name = 'Signal 4'
      | sbobj.Groups.Signals(4).XData = [0 10]
      | sbobj.Groups.Signals(4).YData = [0 0]
  Signal 1 : Outport  Tag=STV Outport
  Signal 2 : Outport  Tag=STV Outport  Port=2
  Signal 3 : Outport  Tag=STV Outport  Port=3
  Signal 4 : Outport  Tag=STV Outport  Port=4
  wires:
  FromWs/1 -> Demux/1
  Demux/1 -> Signal 1/1
  Demux/2 -> Signal 2/1
  Demux/3 -> Signal 3/1
  Demux/4 -> Signal 4/1

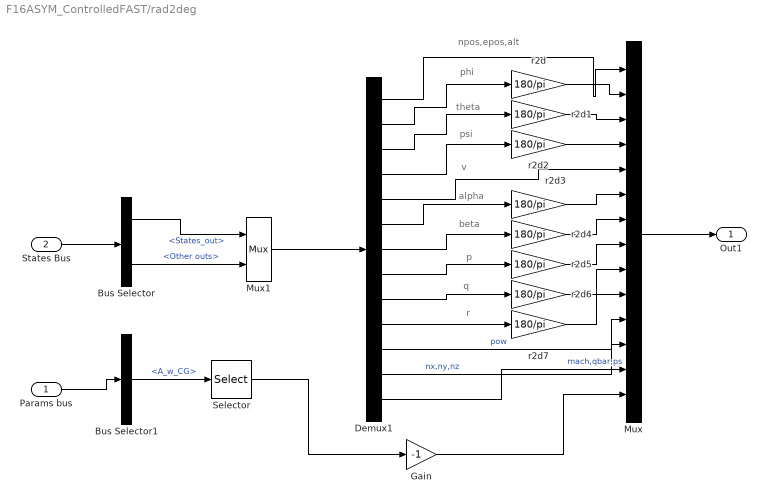
== system F16ASYM_ControlledFAST/rad2deg ==
  note: npos,epos,alt
  note: phi
  note: theta
  note: psi
  note: v
  note: alpha
  note: beta
  note: p
  note: q
  note: r
  Params bus : Inport
  States Bus : Inport  Port=2
  Bus Selector : BusSelector  OutputSignals=States_out,Other outs
  Bus Selector1 : BusSelector  OutputSignals=A_w_CG
  Demux1 : Demux  Outputs=[3 1 1 1 1 1 1 1 1 1 1 3 3]
  Gain : Gain  Gain=-1
  Mux : Mux  Inputs=[3 1 1 1 1 1 1 1 1 1 1 3 3 1]
  Mux1 : Mux  Inputs=2
  Selector : Selector  InputPortWidth=3  IndexOptions=Index vector (dialog)  Indices=3  OutputSizes=1
  r2d{,1..7} (8 alike) : Gain  Gain=180/pi  SaturateOnIntegerOverflow=on  OutDataTypeStr=Inherit: Same as input  ParamDataTypeStr=Inherit: Same as input
  Out1 : Outport
  wires:
  Mux1/1 -> Demux1/1
  Demux1/2 -> r2d/1
  Demux1/3 -> r2d1/1
  Demux1/4 -> r2d2/1
  Demux1/1 -> Mux/1
  Demux1/5 -> Mux/5
  r2d2/1 -> Mux/4
  r2d1/1 -> Mux/3
  r2d/1 -> Mux/2
  Demux1/6 -> r2d3/1
  Demux1/7 -> r2d4/1
  Demux1/8 -> r2d5/1
  Demux1/9 -> r2d6/1
  Demux1/10 -> r2d7/1
  r2d4/1 -> Mux/7
  r2d5/1 -> Mux/8
  r2d6/1 -> Mux/9
  r2d7/1 -> Mux/10
  Mux/1 -> Out1/1
  Demux1/12 -> Mux/12  "nx,ny,nz"
  Demux1/13 -> Mux/13  "mach,qbar,ps"
  r2d3/1 -> Mux/6
  Demux1/11 -> Mux/11  "pow"
  Bus Selector/1 -> Mux1/1  "<States_out>"
  Bus Selector/2 -> Mux1/2  "<Other outs>"
  States Bus/1 -> Bus Selector/1
  Params bus/1 -> Bus Selector1/1
  Bus Selector1/1 -> Selector/1  "<A_w_CG>"
  Selector/1 -> Gain/1
  Gain/1 -> Mux/14

== system F16ASYM_ControlledFAST/Environment params Estimations1/__InputSSForSFun__ ==
  All_meas : Inport
  temporaryBusSelectName_1 : BusSelector  OutputSignals=Alt meas (m),V_TAS (m/s),AoA meas (rad),SS meas (rad),omega_b meas (rad/s),Euler meas (rad),an_b_CG meas (m/s^2),Throttle_meas
  __UniqueOutportName__1__ : Outport
  __UniqueOutportName__2__ : Outport  Port=2
  __UniqueOutportName__3__ : Outport  Port=3
  __UniqueOutportName__4__ : Outport  Port=4
  __UniqueOutportName__5__ : Outport  Port=5
  __UniqueOutportName__6__ : Outport  Port=6
  __UniqueOutportName__7__ : Outport  Port=7
  __UniqueOutportName__8__ : Outport  Port=8
  wires:
  All_meas/1 -> temporaryBusSelectName_1/1
  temporaryBusSelectName_1/1 -> __UniqueOutportName__1__/1  "<Alt meas (m)>"
  temporaryBusSelectName_1/2 -> __UniqueOutportName__2__/1  "<V_TAS (m/s)>"
  temporaryBusSelectName_1/3 -> __UniqueOutportName__3__/1  "<AoA meas (rad)>"
  temporaryBusSelectName_1/4 -> __UniqueOutportName__4__/1  "<SS meas (rad)>"
  temporaryBusSelectName_1/5 -> __UniqueOutportName__5__/1  "<omega_b meas (rad/s)>"
  temporaryBusSelectName_1/6 -> __UniqueOutportName__6__/1  "<Euler meas (rad)>"
  temporaryBusSelectName_1/7 -> __UniqueOutportName__7__/1  "<an_b_CG meas (m/s^2)>"
  temporaryBusSelectName_1/8 -> __UniqueOutportName__8__/1  "<Throttle_meas>"

== system F16ASYM_ControlledFAST/Environment params Estimations1/__OutputSSForSFun__ ==
  __UniqueInportName__1__ : Inport
  __UniqueInportName__2__ : Inport  Port=2
  __UniqueInportName__3__ : Inport  Port=3
  __UniqueInportName__4__ : Inport  Port=4
  __UniqueInportName__5__ : Inport  Port=5
  Mux1 : BusCreator  Inputs=5
  Params : Outport
  wires:
  __UniqueInportName__1__/1 -> Mux1/1  "q (Pa)"
  __UniqueInportName__2__/1 -> Mux1/2  "T_F_b->F_T"
  __UniqueInportName__3__/1 -> Mux1/3  "T_F_b->F_w"
  __UniqueInportName__4__/1 -> Mux1/4  "A_w_CG"
  __UniqueInportName__5__/1 -> Mux1/5  "A_b_CG"
  Mux1/1 -> Params/1

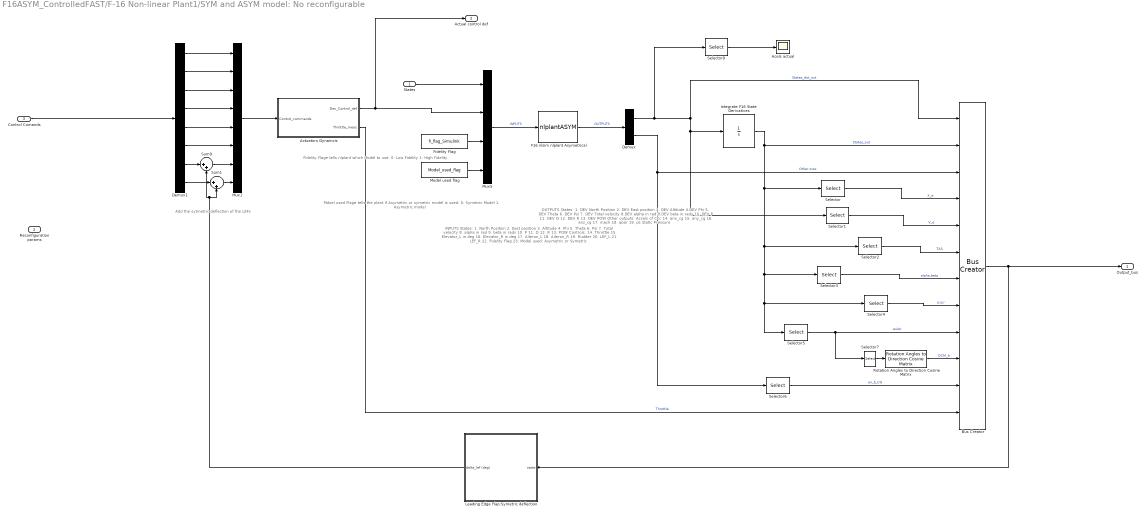
== system F16ASYM_ControlledFAST/F-16 Non-linear Plant1/SYM and ASYM model: No reconfigurable ==
  note: Mdoel used  Flage tells the plant
      |  if Asymetric or symetric model is used:
      | 0: Symetric Model
      | 1: Asymetric model
  note: INPUTS
      | States:
      | 1. North Position
      | 2. East position
      | 3. Altitude
      | 4. Phi
      | 5. Theta
      | 6. Psi
      | 7. Total velocity
      | 8. alpha in rad
      | 9. beta in rads
      | 10. P
      | 11. Q
      | 12. R
      | 13. POW
      |
      | Controls:
      | 14. Throttle
      | 15. Elevator_L in deg
      | 16. Elevator_R in deg
      | 17. Aileron_L
      | 18. Aileron_R
      | 19. Rudder
      | 20. LEF_L
      | 21. LEF_R
      |
      | 22. Fidelity Flag
      |
      | 23. Model used: Asymetric or Symetric
  note: Fidelity Flage tells nlplant
      | which Model to use:
      | 0: Low Fidelity
      | 1: High Fidelity
  note: OUTPUTS
      | States:
      | 1. DEV North Position
      | 2. DEV East position
      | 3. DEV Altitude
      | 4.DEV  Phi
      | 5. DEV Theta
      | 6. DEV Psi
      | 7. DEV Total velocity
      | 8.DEV alpha in rad
      | 9.DEV  beta in rads
      | 10. DEV P
      | 11. DEV Q
      | 12. DEV R
      | 13. DEV POW
      |
      | Other outputs:
      | Accels of CG:
      | 14. anx_cg
      | 15. any_cg
      | 16. anz_cg
      | 17. mach
      | 18. qbar
      | 19. ps   Static Pressure
  note: Add the sytmetric deflection of the LEFs
  States : Inport
  Reconfiguration params : Inport  Port=2
  Control Comands : Inport  Port=3
  Acels actual : Scope
      settings: YMin=-0.04  YMax=0.09  SaveName=ScopeData14
  Actuators Dynamcis : Subsystem  TreatAsAtomicUnit=on
  Bus Creator : BusCreator  Inputs=12
  Demux : Demux  Outputs=[13 6]
  Demux1 : Demux  Outputs=8
  F16 nlsim nlplant Asymetrical : MATLABFcn  MATLABFcn=nlplantASYM  OutputDimensions=19  OutputSignalType=real
  Fidelity Flag : Constant  Value=fi_flag_Simulink
  Integrate F16 State Derivatives : Integrator  InitialCondition=trim_state
  Leading Edge Flap:Symetric deflection : Subsystem
  Model used flag : Constant  Value=Model_used_flag
  Mux1 : Mux  Inputs=8
  Mux5 : Mux  Inputs=[13 8 1 1]
  Rotation Angles to Direction Cosine Matrix : aerolibtransform2/Rotation Angles to Direction Cosine Matrix  rotationOrder=ZYX
  Selector : Selector  InputPortWidth=13  IndexOptions=Index vector (dialog)  Indices=[1:3]  OutputSizes=1
  Selector1 : Selector  InputPortWidth=13  IndexOptions=Index vector (dialog)  Indices=[1:3]  OutputSizes=1
  Selector2 : Selector  InputPortWidth=13  IndexOptions=Index vector (dialog)  Indices=[7]  OutputSizes=1
  Selector3 : Selector  InputPortWidth=13  IndexOptions=Index vector (dialog)  Indices=[8:9]  OutputSizes=1
  Selector4 : Selector  InputPortWidth=13  IndexOptions=Index vector (dialog)  Indices=[10:12]  OutputSizes=1
  Selector5 : Selector  InputPortWidth=13  IndexOptions=Index vector (dialog)  Indices=[4:6]  OutputSizes=1
  Selector6 : Selector  InputPortWidth=6  IndexOptions=Index vector (dialog)  Indices=[1:3]  OutputSizes=1
  Selector7 : Selector  InputPortWidth=3  IndexOptions=Index vector (dialog)  Indices=[3 2 1]  OutputSizes=1
  Selector9 : Selector  InputPortWidth=13  IndexOptions=Index vector (dialog)  Indices=[10:12]  OutputSizes=1
  Sum1 : Sum  Inputs=|++  SaturateOnIntegerOverflow=on  InputSameDT=on  OutDataTypeStr=Inherit: Same as first input
  Sum9 : Sum  Inputs=|++  SaturateOnIntegerOverflow=on  InputSameDT=on  OutDataTypeStr=Inherit: Same as first input
  Output_bus : Outport
  Actual control def : Outport  Port=2
  wires:
  Selector7/1 -> Rotation Angles to Direction Cosine Matrix/1
  Demux/2 -> Bus Creator/3, Selector6/1  "Other outs"
  Selector6/1 -> Bus Creator/11  "an_b_CG"
  Selector5/1 -> Bus Creator/9, Selector7/1  "euler"
  Selector4/1 -> Bus Creator/8  "p,q,r"
  Selector3/1 -> Bus Creator/7  "alpha,beta"
  Selector2/1 -> Bus Creator/6  "TAS"
  Selector1/1 -> Bus Creator/5  "V_e"
  Selector/1 -> Bus Creator/4  "X_e"
  Demux/1 -> Integrate F16 State Derivatives/1, Selector1/1, Bus Creator/1, Selector9/1  "States_dot_out"
  Actuators Dynamcis/2(Throttle_meas) -> Bus Creator/12  "Throttle"
  Selector9/1 -> Acels actual/1
  Mux1/1 -> Actuators Dynamcis/1(Control_commands)
  Sum1/1 -> Mux1/8
  Sum9/1 -> Mux1/7
  Demux1/6 -> Mux1/6
  Demux1/4 -> Mux1/4
  Demux1/2 -> Mux1/2
  Demux1/1 -> Mux1/1
  Demux1/3 -> Mux1/3
  Demux1/5 -> Mux1/5
  Leading Edge Flap:Symetric deflection/1(delta_lef (deg)) -> Sum9/2, Sum1/2
  Demux1/7 -> Sum9/1
  Demux1/8 -> Sum1/1
  Model used flag/1 -> Mux5/4
  Actuators Dynamcis/1(Dec_Control_def) -> Mux5/2, Actual control def/1
  F16 nlsim nlplant Asymetrical/1 -> Demux/1  "OUTPUTS"
  Mux5/1 -> F16 nlsim nlplant Asymetrical/1  "INPUTS"
  States/1 -> Mux5/1
  Control Comands/1 -> Demux1/1
  Fidelity Flag/1 -> Mux5/3
  Bus Creator/1 -> Leading Edge Flap:Symetric deflection/1(state), Output_bus/1
  Rotation Angles to Direction Cosine Matrix/1 -> Bus Creator/10  "DCM_b"
  Integrate F16 State Derivatives/1 -> Bus Creator/2, Selector/1, Selector2/1, Selector3/1, Selector4/1, Selector5/1  "States_out"

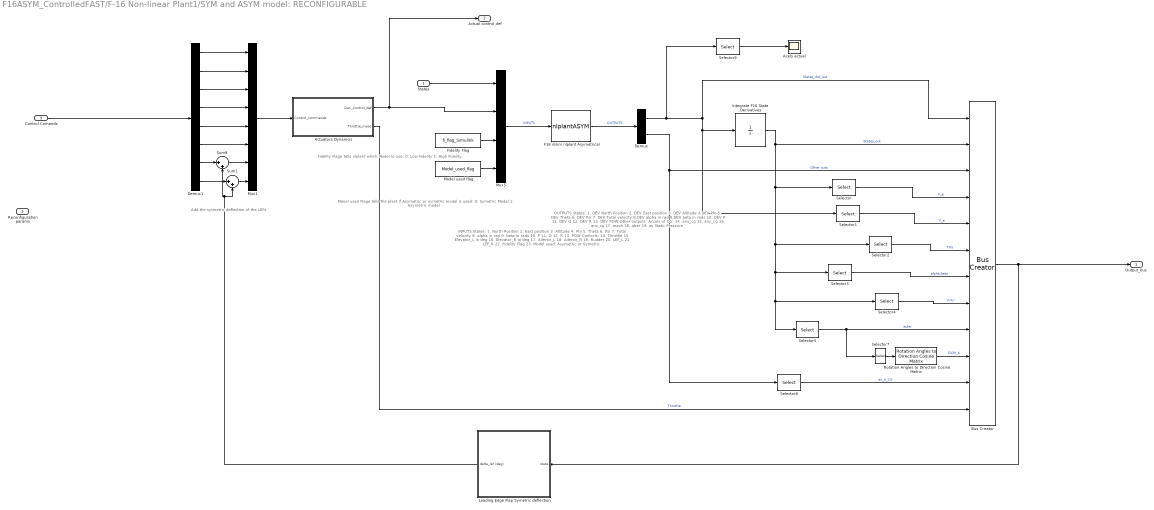
== system F16ASYM_ControlledFAST/F-16 Non-linear Plant1/SYM and ASYM model: RECONFIGURABLE ==
  note: Add the sytmetric deflection of the LEFs
  note: OUTPUTS
      | States:
      | 1. DEV North Position
      | 2. DEV East position
      | 3. DEV Altitude
      | 4.DEV  Phi
      | 5. DEV Theta
      | 6. DEV Psi
      | 7. DEV Total velocity
      | 8.DEV alpha in rad
      | 9.DEV  beta in rads
      | 10. DEV P
      | 11. DEV Q
      | 12. DEV R
      | 13. DEV POW
      |
      | Other outputs:
      | Accels of CG:
      | 14. anx_cg
      | 15. any_cg
      | 16. anz_cg
      | 17. mach
      | 18. qbar
      | 19. ps   Static Pressure
  note: Fidelity Flage tells nlplant
      | which Model to use:
      | 0: Low Fidelity
      | 1: High Fidelity
  note: INPUTS
      | States:
      | 1. North Position
      | 2. East position
      | 3. Altitude
      | 4. Phi
      | 5. Theta
      | 6. Psi
      | 7. Total velocity
      | 8. alpha in rad
      | 9. beta in rads
      | 10. P
      | 11. Q
      | 12. R
      | 13. POW
      |
      | Controls:
      | 14. Throttle
      | 15. Elevator_L in deg
      | 16. Elevator_R in deg
      | 17. Aileron_L
      | 18. Aileron_R
      | 19. Rudder
      | 20. LEF_L
      | 21. LEF_R
      |
      | 22. Fidelity Flag
      |
      | 23. Model used: Asymetric or Symetric
  note: Mdoel used  Flage tells the plant
      |  if Asymetric or symetric model is used:
      | 0: Symetric Model
      | 1: Asymetric model
  States : Inport
  Reconfiguration params : Inport  Port=2
  Control Comands : Inport  Port=3
  Acels actual : Scope
      settings: YMin=-0.04  YMax=0.09  SaveName=ScopeData14
  Actuators Dynamcis : Subsystem  TreatAsAtomicUnit=on
  Bus Creator : BusCreator  Inputs=12
  Demux : Demux  Outputs=[13 6]
  Demux1 : Demux  Outputs=8
  F16 nlsim nlplant Asymetrical : MATLABFcn  MATLABFcn=nlplantASYM  OutputDimensions=19  OutputSignalType=real
  Fidelity Flag : Constant  Value=fi_flag_Simulink
  Integrate F16 State Derivatives : Integrator  InitialCondition=trim_state
  Leading Edge Flap:Symetric deflection : Subsystem
  Model used flag : Constant  Value=Model_used_flag
  Mux1 : Mux  Inputs=8
  Mux5 : Mux  Inputs=[13 8 1 1]
  Rotation Angles to Direction Cosine Matrix : aerolibtransform2/Rotation Angles to Direction Cosine Matrix  rotationOrder=ZYX
  Selector : Selector  InputPortWidth=13  IndexOptions=Index vector (dialog)  Indices=[1:3]  OutputSizes=1
  Selector1 : Selector  InputPortWidth=13  IndexOptions=Index vector (dialog)  Indices=[1:3]  OutputSizes=1
  Selector2 : Selector  InputPortWidth=13  IndexOptions=Index vector (dialog)  Indices=[7]  OutputSizes=1
  Selector3 : Selector  InputPortWidth=13  IndexOptions=Index vector (dialog)  Indices=[8:9]  OutputSizes=1
  Selector4 : Selector  InputPortWidth=13  IndexOptions=Index vector (dialog)  Indices=[10:12]  OutputSizes=1
  Selector5 : Selector  InputPortWidth=13  IndexOptions=Index vector (dialog)  Indices=[4:6]  OutputSizes=1
  Selector6 : Selector  InputPortWidth=6  IndexOptions=Index vector (dialog)  Indices=[1:3]  OutputSizes=1
  Selector7 : Selector  InputPortWidth=3  IndexOptions=Index vector (dialog)  Indices=[3 2 1]  OutputSizes=1
  Selector9 : Selector  InputPortWidth=13  IndexOptions=Index vector (dialog)  Indices=[10:12]  OutputSizes=1
  Sum1 : Sum  Inputs=|++  SaturateOnIntegerOverflow=on  InputSameDT=on  OutDataTypeStr=Inherit: Same as first input
  Sum9 : Sum  Inputs=|++  SaturateOnIntegerOverflow=on  InputSameDT=on  OutDataTypeStr=Inherit: Same as first input
  Output_bus : Outport
  Actual control def : Outport  Port=2
  wires:
  Integrate F16 State Derivatives/1 -> Selector5/1, Selector4/1, Selector3/1, Selector2/1, Selector/1, Bus Creator/2  "States_out"
  Rotation Angles to Direction Cosine Matrix/1 -> Bus Creator/10  "DCM_b"
  Bus Creator/1 -> Output_bus/1, Leading Edge Flap:Symetric deflection/1(state)
  Fidelity Flag/1 -> Mux5/3
  Control Comands/1 -> Demux1/1
  States/1 -> Mux5/1
  Mux5/1 -> F16 nlsim nlplant Asymetrical/1  "INPUTS"
  F16 nlsim nlplant Asymetrical/1 -> Demux/1  "OUTPUTS"
  Actuators Dynamcis/1(Dec_Control_def) -> Actual control def/1, Mux5/2
  Model used flag/1 -> Mux5/4
  Demux1/8 -> Sum1/1
  Demux1/7 -> Sum9/1
  Leading Edge Flap:Symetric deflection/1(delta_lef (deg)) -> Sum1/2, Sum9/2
  Demux1/5 -> Mux1/5
  Demux1/3 -> Mux1/3
  Demux1/1 -> Mux1/1
  Demux1/2 -> Mux1/2
  Demux1/4 -> Mux1/4
  Demux1/6 -> Mux1/6
  Sum9/1 -> Mux1/7
  Sum1/1 -> Mux1/8
  Mux1/1 -> Actuators Dynamcis/1(Control_commands)
  Selector9/1 -> Acels actual/1
  Actuators Dynamcis/2(Throttle_meas) -> Bus Creator/12  "Throttle"
  Demux/1 -> Selector9/1, Bus Creator/1, Selector1/1, Integrate F16 State Derivatives/1  "States_dot_out"
  Selector/1 -> Bus Creator/4  "X_e"
  Selector1/1 -> Bus Creator/5  "V_e"
  Selector2/1 -> Bus Creator/6  "TAS"
  Selector3/1 -> Bus Creator/7  "alpha,beta"
  Selector4/1 -> Bus Creator/8  "p,q,r"
  Selector5/1 -> Selector7/1, Bus Creator/9  "euler"
  Selector6/1 -> Bus Creator/11  "an_b_CG"
  Demux/2 -> Selector6/1, Bus Creator/3  "Other outs"
  Selector7/1 -> Rotation Angles to Direction Cosine Matrix/1
